simulink model "Single_Phase_Fully_Controlled_Converter_fed_DC_Moter_Drive"  (R2020b)
settings: Solver=VariableStepAuto  StartTime=0.0  StopTime=10  RelTol=1e-3
libraries: powerlib x9, eeStairGenerator x1
settings Model: Creator=adima  LastModifiedBy=adima

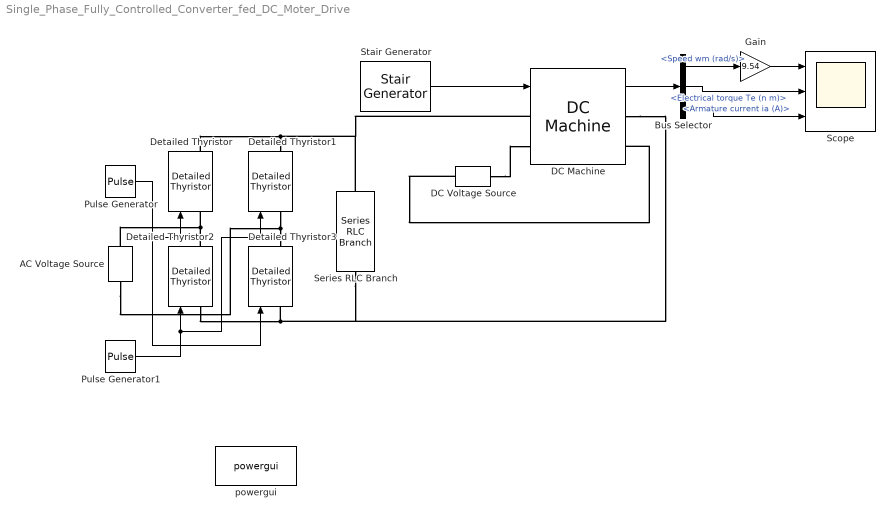
== system Single_Phase_Fully_Controlled_Converter_fed_DC_Moter_Drive ==
  AC Voltage Source : powerlib/Electrical Sources/AC Voltage Source  Amplitude=230  Phase=0  Frequency=50  SampleTime=0  Measurements=None  BusType=swing  Pref=10e3  Qref=0  Qmin=-inf  Qmax=+inf
  Bus Selector : BusSelector  OutputSignals=Speed wm (rad/s),Electrical torque Te (n m),Armature current ia (A)
  DC Machine : powerlib/Machines/DC Machine  PresetModel=01: 5HP 240V 1750RPM Field:300V  MechanicalLoad=Torque TL  FieldType=Wound  ShowDetailedParameters=on  MeasurementBus=off  RLa=[2.581 0.028]  RLf=[281.3 156]  Laf=0.9483  MachineConstant=Torque constant (N.m/A)  Ke=1.8  Kt=1.8  J=0.02215  Bm=0.002953  Tf=0.5161  w0=1  Ifinit=1.06647706944812  TsPowergui=0  TsBlock=-1
  DC Voltage Source : powerlib/Electrical Sources/DC Voltage Source  Amplitude=300  Measurements=None
  Detailed Thyristor{,1..3} (4 alike) : powerlib/Power Electronics/Detailed Thyristor  Ron=0.001  Lon=1e-3  Vf=0.8  IL=0.1  Tq=100e-6  IC=0  Rs=500  Cs=250e-9  Measurements=on
      settings: SourceProductBaseCode=PS
  Gain : Gain  Gain=9.54
  Pulse Generator : DiscretePulseGenerator  PulseType=Time based  Period=1/50  PulseWidth=30  PhaseDelay=30*((20e-3)/360)
  Pulse Generator1 : DiscretePulseGenerator  PulseType=Time based  Period=1/50  PulseWidth=30  PhaseDelay=210*((20e-3)/360)
  Scope : Scope  NumInputPorts=3
  Series RLC Branch : powerlib/Elements/Series RLC Branch  LConnTagsString=__new0  RConnTagsString=__new0  BranchType=R  Resistance=1  Inductance=1e-3  SetiL0=off  InitialCurrent=0  Capacitance=1e-6  Setx0=off  InitialVoltage=0  Measurements=None
  Stair Generator : eeStairGenerator/Stair Generator  LabelModeActiveChoice=Discrete  TimeInput=[0 3 5 10]  AmplitudeInput=[0 5.075 10.15 20.3]  SampleTime=-1  RepeatPattern=off  OutDataTypeStr=double
      settings: SourceProductBaseCode=PS
  powergui : powerlib/powergui  Priority=1  SimulationMode=Discrete  SampleTime=5e-6  frequency=60  Iterations=50  frequencyindice=50  Pbase=100e6  ErrMax=1e-4  UnitsV=kV  UnitsW=MW  buscounter=0  FunctionMessages=off  echomessages=off  EnableUseOfTLC=off  CurrentSourceSwitches=off  DisableSnubberDevices=off  DisableRonSwitches=off  DisableVfSwitches=off  DisplayEquations=off  AutomaticDiscreteSolvers=off  SolverType=Tustin/Backward Euler (TBE)  Interpol=off  ExternalGateDelay=off  methode=off  Ts=100  x0status=blocks  SPID=on  SwTol=0  HookPort=off  NonlinearTolerance=1e-4  nMaxIteration=100  ContinueOnMaxIteration=off  RestoreLinks=warning  ResistiveCurrentMeasurement=off  Frange=[0:2:500]  Ylog=off  Xlog=on  ShowGrid=off  save=off  variable=ZData  structure=0  ZoomFFT=off  StartTime=0.0  cycles=1  DisplayStyle=1  fundamental=60  FreqAxis=off  MaxFrequency=1000  frequencyindicesteady=1  RmsSteady=1  display=off
  wires:
  Stair Generator/1 -> DC Machine/1
  DC Machine/1 -> Bus Selector/1
  Bus Selector/2 -> Scope/2  "<Electrical torque Te (n m)>"
  Pulse Generator1/1 -> Detailed Thyristor1/1, Detailed Thyristor2/1
  Pulse Generator/1 -> Detailed Thyristor/1, Detailed Thyristor3/1
  Bus Selector/3 -> Scope/3  "<Armature current ia (A)>"
  Gain/1 -> Scope/1
  Bus Selector/1 -> Gain/1  "<Speed wm (rad/s)>"
  connections:
  DC Voltage Source/RConn1 -- DC Machine/LConn2
  DC Voltage Source/LConn1 -- DC Machine/RConn2
  Detailed Thyristor2/RConn1 -- AC Voltage Source/RConn1 -- Detailed Thyristor/LConn1
  Detailed Thyristor/RConn1 -- Series RLC Branch/LConn1 -- DC Machine/LConn1 -- Detailed Thyristor1/RConn1
  Detailed Thyristor1/LConn1 -- AC Voltage Source/LConn1 -- Detailed Thyristor3/RConn1
  Detailed Thyristor2/LConn1 -- Series RLC Branch/RConn1 -- DC Machine/RConn1 -- Detailed Thyristor3/LConn1
